simulink model "onlySF1"  (R2018b)
settings: Solver=VariableStepAuto  StartTime=0.0  StopTime=60  RelTol=1e-3
settings Model: Creator=jinwooro  LastModifiedBy=jinwooro

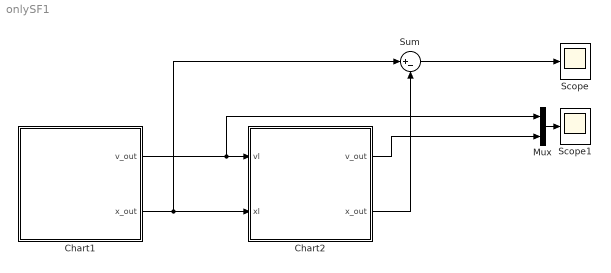
== system onlySF1 ==
  Chart1 : Stateflow chart  TreatAsAtomicUnit=on
  Chart2 : Stateflow chart  TreatAsAtomicUnit=on
  Mux : Mux  Inputs=2
  Scope : Scope
  Scope1 : Scope
  Sum : Sum  Inputs=|+-
  wires:
  Chart1/1(v_out) -> Mux/1, Chart2/1(vl)
  Chart1/2(x_out) -> Sum/1, Chart2/2(xl)
  Sum/1 -> Scope/1
  Chart2/2(x_out) -> Sum/2
  Mux/1 -> Scope1/1
  Chart2/1(v_out) -> Mux/2

== stateflow chart onlySF1/Chart2 ==
  settings: updateMethod=CONTINUOUS
  state LocB
    du:
    v_dot = 0;
    x_dot = 0;
    v_out = v;
    x_out = x;
  state LocA
    du:
    v_dot = 0.9 * (vl-v);
    x_dot = v;
    v_out = v;
    x_out = x;
  (default) -> LocA : {x = -25;
      | v = 0;}
  LocA -> LocB : [power(xl - x, 0.5) < 0]{v = 0;}
  data: v_out output; vl input; x_out output; v local; x local; xl input
  data vl settings: updateMethod=SF_CONTINUOUS_TIME_DATA
  data v settings: updateMethod=SF_CONTINUOUS_TIME_DATA
  data x settings: updateMethod=SF_CONTINUOUS_TIME_DATA
  data xl settings: updateMethod=SF_CONTINUOUS_TIME_DATA

== stateflow chart onlySF1/Chart1 ==
  settings: updateMethod=CONTINUOUS
  state LocB
    en:
    v = 25;
    du:
    v_dot = -2;
    x_dot = v;
    v_out = v;
    x_out = x;
  state LocA
    du:
    v_dot = 2;
    x_dot = v;
    v_out = v;
    x_out = x;
  (default) -> LocA : {x = 0;
      | v= 0;}
  LocA -> LocB : [v >= 25]
  LocB -> LocA : [v <= 13]
  data: v_out output; x local; x_out output; v local
  data x settings: updateMethod=SF_CONTINUOUS_TIME_DATA
  data v settings: updateMethod=SF_CONTINUOUS_TIME_DATA
